simulink model "T3_SIM2"  (R2023b)
settings: Solver=VariableStepAuto  StartTime=0.0  StopTime=20  RelTol=1e-3
undefined symbols (not defined in the file): A_1, A_10, A_11, A_12, A_2, A_3, A_4, A_5, A_6, A_7, A_8, A_9, B_1, B_10, B_11, B_12, B_2, B_3, B_4, B_5, B_6, B_7, B_8, B_9, C_1, C_10, C_11, C_12, C_2, C_3, C_4, C_5, C_6, C_7, C_8, C_9, D_1, D_10, D_11, D_12, D_2, D_3, D_4, D_5, D_6, D_7, D_8, D_9, u1_12
settings Model: Creator=Mihai Dinu  LastModifiedBy=Mihai Dinu

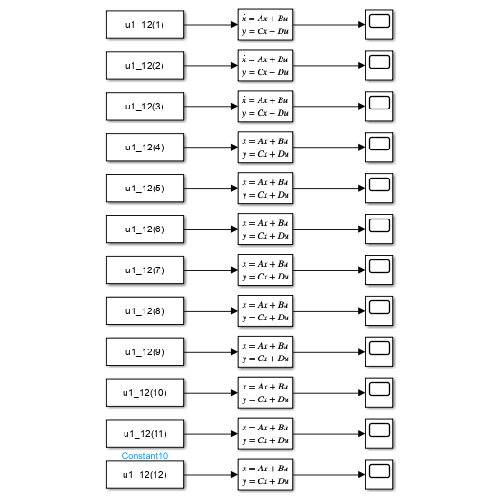
[thumbnail: Simulink's stored preview of the top-level diagram]
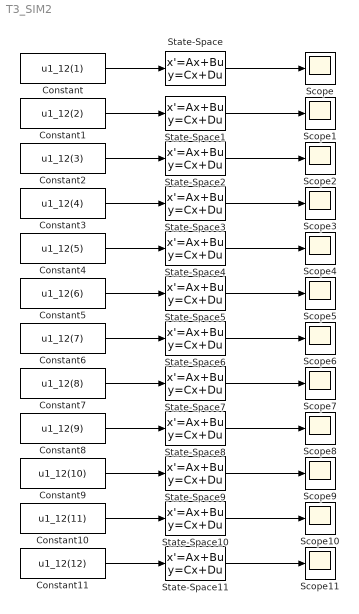
== system T3_SIM2 ==
  Constant : Constant  Value=u1_12(1)
  Constant1 : Constant  Value=u1_12(2)
  Constant10 : Constant  Value=u1_12(11)
  Constant11 : Constant  Value=u1_12(12)
  Constant2 : Constant  Value=u1_12(3)
  Constant3 : Constant  Value=u1_12(4)
  Constant4 : Constant  Value=u1_12(5)
  Constant5 : Constant  Value=u1_12(6)
  Constant6 : Constant  Value=u1_12(7)
  Constant7 : Constant  Value=u1_12(8)
  Constant8 : Constant  Value=u1_12(9)
  Constant9 : Constant  Value=u1_12(10)
  Scope{,1..11} (12 alike) : Scope
  State-Space : StateSpace  A=A_1  B=B_1  C=C_1  D=D_1  InitialCondition=0
  State-Space1 : StateSpace  A=A_2  B=B_2  C=C_2  D=D_2  InitialCondition=0
  State-Space10 : StateSpace  A=A_11  B=B_11  C=C_11  D=D_11  InitialCondition=0
  State-Space11 : StateSpace  A=A_12  B=B_12  C=C_12  D=D_12  InitialCondition=0
  State-Space2 : StateSpace  A=A_3  B=B_3  C=C_3  D=D_3  InitialCondition=0
  State-Space3 : StateSpace  A=A_4  B=B_4  C=C_4  D=D_4  InitialCondition=0
  State-Space4 : StateSpace  A=A_5  B=B_5  C=C_5  D=D_5  InitialCondition=0
  State-Space5 : StateSpace  A=A_6  B=B_6  C=C_6  D=D_6  InitialCondition=0
  State-Space6 : StateSpace  A=A_7  B=B_7  C=C_7  D=D_7  InitialCondition=0
  State-Space7 : StateSpace  A=A_8  B=B_8  C=C_8  D=D_8  InitialCondition=0
  State-Space8 : StateSpace  A=A_9  B=B_9  C=C_9  D=D_9  InitialCondition=0
  State-Space9 : StateSpace  A=A_10  B=B_10  C=C_10  D=D_10  InitialCondition=0
  wires:
  Constant/1 -> State-Space/1
  State-Space/1 -> Scope/1
  Constant1/1 -> State-Space1/1
  State-Space1/1 -> Scope1/1
  Constant2/1 -> State-Space2/1
  State-Space2/1 -> Scope2/1
  Constant3/1 -> State-Space3/1
  State-Space3/1 -> Scope3/1
  Constant5/1 -> State-Space5/1
  Constant4/1 -> State-Space4/1
  State-Space6/1 -> Scope6/1
  Constant6/1 -> State-Space6/1
  State-Space7/1 -> Scope7/1
  State-Space4/1 -> Scope4/1
  Constant7/1 -> State-Space7/1
  State-Space5/1 -> Scope5/1
  Constant9/1 -> State-Space9/1
  Constant8/1 -> State-Space8/1
  State-Space10/1 -> Scope10/1
  Constant10/1 -> State-Space10/1
  State-Space11/1 -> Scope11/1
  State-Space8/1 -> Scope8/1
  Constant11/1 -> State-Space11/1
  State-Space9/1 -> Scope9/1
